simulink library "CA_library"  (R2017b)
settings: Solver=VariableStepAuto  StartTime=0.0  StopTime=10.0  RelTol=1e-3
undefined symbols (not defined in the file or in its folder): B2
libraries: dspmtrx3 x5, dspinverses x1
settings Model: Creator=Liam Uni  LastModifiedBy=Liam Uni

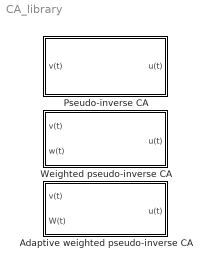
== system CA_library ==
  Adaptive weighted pseudo-inverse CA : Subsystem  mask{B2=B2}
      mask DialogControl DescGroupVar Prompt: Adaptive weighted pseudo-inverse CA
      mask DialogControl DescTextVar Prompt: Control allocation module using the adaptive control allocation method. The input W(t) is a vector of the diagonal elements of W
      mask Display:
      | disp('Adaptive')
      | 
      | port_label('input', 1, 'v(t)');
      | port_label('input', 2, 'W(t)');
      | port_label('output', 1, 'u(t)');
  Pseudo-inverse CA : Subsystem  mask{B2=B2}
      mask DialogControl DescGroupVar Prompt: Pseudo-inverse CA
      mask DialogControl DescTextVar Prompt: Control allocation module using the pinv() function.
      mask Display:
      | disp('B^+')
      | port_label('input', 1, 'v(t)');
      | port_label('output', 1, 'u(t)');
  Weighted pseudo-inverse CA : Subsystem  mask{B2=B2}
      mask DialogControl DescGroupVar Prompt: Weighted pseudo-inverse CA
      mask DialogControl DescTextVar Prompt: Control allocation module using the weighted Moore-Penrose inverse B^+=WB'(BWB')^-1. The input W(t) is a vector of the diagonal elements of W.
      mask Display:
      | disp('WB(BWB)^-1')
      | port_label('input', 1, 'v(t)');
      | port_label('input', 2, 'W(t)');
      | port_label('output', 1, 'u(t)');

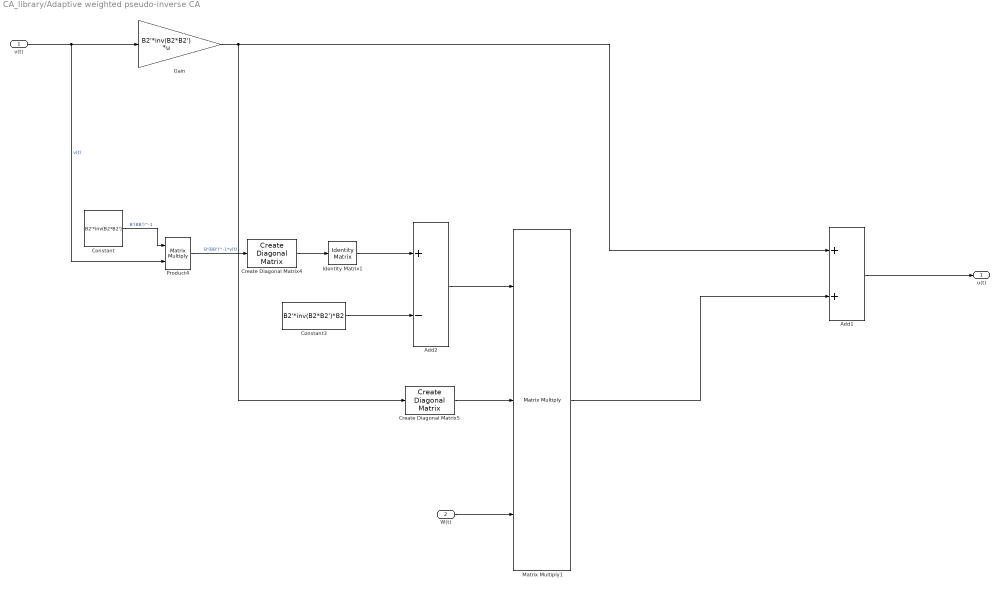
== system CA_library/Adaptive weighted pseudo-inverse CA ==
  v(t) : Inport
  W(t) : Inport  Port=2
  Add1 : Sum
  Add2 : Sum  Inputs=+-
  Constant : Constant  Value=B2'*inv(B2*B2')
  Constant3 : Constant  Value=B2'*inv(B2*B2')*B2
  Create Diagonal Matrix4 : dspmtrx3/Create Diagonal Matrix
      settings: SourceProductName=DSP System Toolbox  SourceProductBaseCode=DS
  Create Diagonal Matrix5 : dspmtrx3/Create Diagonal Matrix
      settings: SourceProductName=DSP System Toolbox  SourceProductBaseCode=DS
  Gain : Gain  Gain=B2'*inv(B2*B2')  Multiplication=Matrix(K*u) (u vector)
  Identity Matrix1 : dspmtrx3/Identity Matrix  Inherit=on  N=5  Ts=1  dataType=double  isSigned=on  wordLen=16  udDataType=sfix(16)  fracBitsMode=Best precision  numFracBits=15  OutDataTypeStr=double  LastOutDataTypeStr=double
      settings: SourceProductName=DSP System Toolbox
  Matrix Multiply1 : Product  Inputs=3  Multiplication=Matrix(*)
  Product4 : Product  Multiplication=Matrix(*)
  u(t) : Outport
  wires:
  v(t)/1 -> Gain/1, Product4/2  "v(t)"
  Gain/1 -> Create Diagonal Matrix5/1, Add1/1
  Product4/1 -> Create Diagonal Matrix4/1  "B'(BB')^-1*v(t)"
  Constant/1 -> Product4/1  "B'(BB')^-1"
  Create Diagonal Matrix4/1 -> Identity Matrix1/1
  Identity Matrix1/1 -> Add2/1
  Constant3/1 -> Add2/2
  Add2/1 -> Matrix Multiply1/1
  Create Diagonal Matrix5/1 -> Matrix Multiply1/2
  Matrix Multiply1/1 -> Add1/2
  Add1/1 -> u(t)/1
  W(t)/1 -> Matrix Multiply1/3

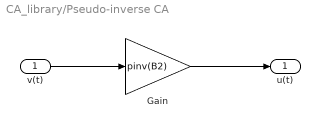
== system CA_library/Pseudo-inverse CA ==
  v(t) : Inport
  Gain : Gain  Gain=pinv(B2)
  u(t) : Outport
  wires:
  v(t)/1 -> Gain/1
  Gain/1 -> u(t)/1

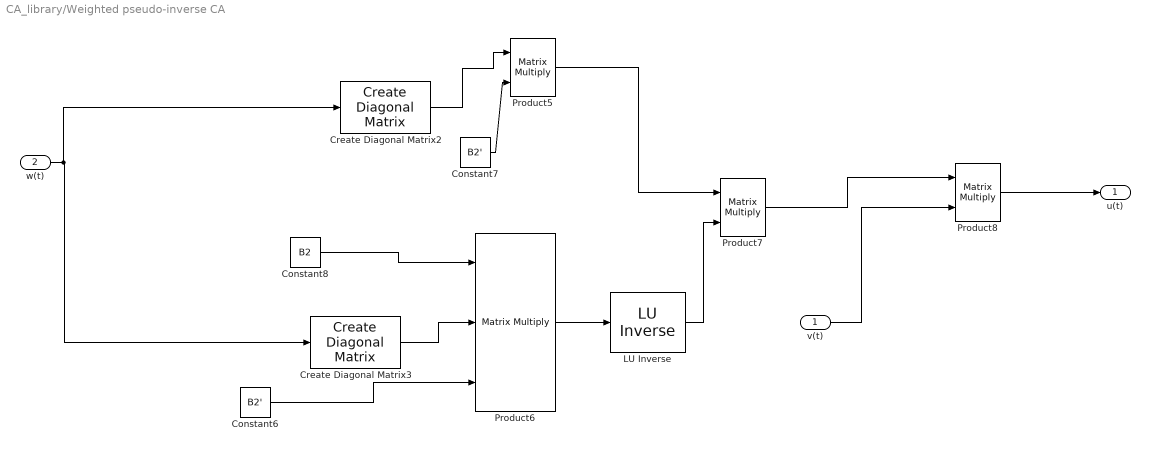
== system CA_library/Weighted pseudo-inverse CA ==
  v(t) : Inport
  w(t) : Inport  Port=2
  " LU Inverse" : dspinverses/ LU Inverse
      settings: SourceProductName=DSP System Toolbox
  Constant6 : Constant  Value=B2'
  Constant7 : Constant  Value=B2'
  Constant8 : Constant  Value=B2
  Create Diagonal Matrix2 : dspmtrx3/Create Diagonal Matrix
      settings: SourceProductName=DSP System Toolbox  SourceProductBaseCode=DS
  Create Diagonal Matrix3 : dspmtrx3/Create Diagonal Matrix
      settings: SourceProductName=DSP System Toolbox  SourceProductBaseCode=DS
  Product5 : Product  Multiplication=Matrix(*)
  Product6 : Product  Inputs=3  Multiplication=Matrix(*)
  Product7 : Product  Multiplication=Matrix(*)
  Product8 : Product  Multiplication=Matrix(*)
  u(t) : Outport
  wires:
  Product8/1 -> u(t)/1
  " LU Inverse"/1 -> Product7/2
  Product6/1 -> " LU Inverse"/1
  Product5/1 -> Product7/1
  Constant7/1 -> Product5/2
  Product7/1 -> Product8/1
  w(t)/1 -> Create Diagonal Matrix2/1, Create Diagonal Matrix3/1
  Create Diagonal Matrix2/1 -> Product5/1
  Constant6/1 -> Product6/3
  Constant8/1 -> Product6/1
  Create Diagonal Matrix3/1 -> Product6/2
  v(t)/1 -> Product8/2
